simulink model "Task_1"  (R2022a)
settings: Solver=VariableStepAuto  StartTime=0.0  StopTime=t_in(end) + 1  FixedStep=t_step  MaxStep=t_step  RelTol=1e-3
settings Model: Creator=jpcas  LastModifiedBy=jpcas

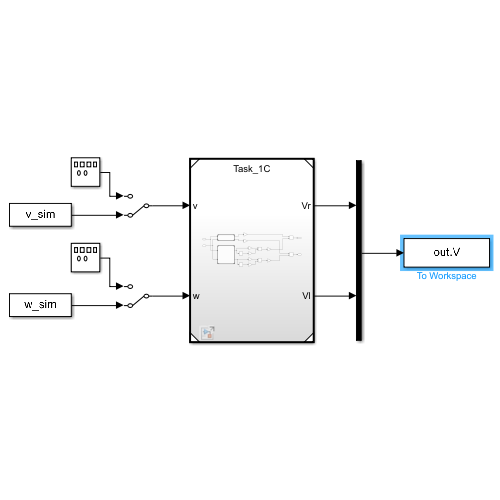
[thumbnail: Simulink's stored preview of the top-level diagram]
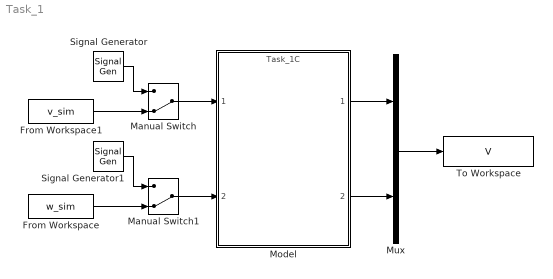
== system Task_1 ==
  From Workspace : FromWorkspace  VariableName=w_sim
  From Workspace1 : FromWorkspace  VariableName=v_sim
  Manual Switch : ManualSwitch  CurrentSetting=0
  Manual Switch1 : ManualSwitch  CurrentSetting=0
  Model : ModelReference  ModelNameDialog=Task_1C  SimulationMode=Normal  ModelReferenceVersion=1.6
  Mux : Mux  Inputs=2
  Signal Generator : SignalGenerator  Units=rad/sec
  Signal Generator1 : SignalGenerator  Units=rad/sec
  To Workspace : ToWorkspace  VariableName=V  SaveFormat=Timeseries  SampleTime=-1
  wires:
  Manual Switch/1 -> Model/1
  Signal Generator/1 -> Manual Switch/1
  Manual Switch1/1 -> Model/2
  Signal Generator1/1 -> Manual Switch1/1
  From Workspace1/1 -> Manual Switch/2
  From Workspace/1 -> Manual Switch1/2
  Model/1 -> Mux/1
  Model/2 -> Mux/2
  Mux/1 -> To Workspace/1
